simulink model "model_2D"  (R2021b)
settings: Solver=VariableStepAuto  StartTime=0.0  StopTime=discretization_time  RelTol=1e-3
values from neighbouring files (symbols this model uses):
  state = current_state+[0.5*time_step^2*input+current_state(2)*time_step,time_step*input]    [Model_1D.m]    (also in Model_der_1D.m = [1,time_step;0,1]; Model_der_2D.m = [1,0,-sin(current_state(3))*0.5*(current_state(5)+current_st; Model_obs_1D.m = [1,0;0,1]; Model_obs_2D.m = [1,0,0,0,0;0,1,0,0,0;0,0,1,0,0;0,0,0,1,0;0,0,0,0,1])
settings Model: Creator=filip  LastModifiedBy=filip

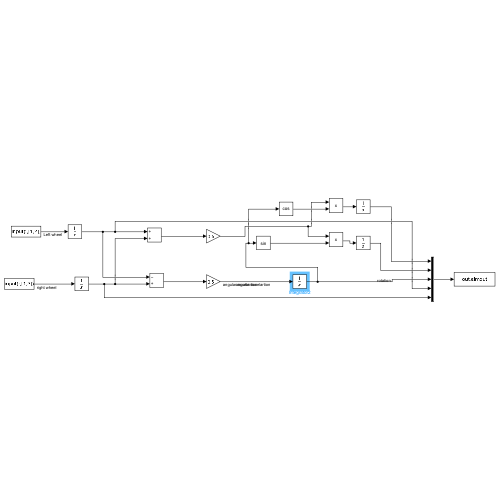
[thumbnail: Simulink's stored preview of the top-level diagram]
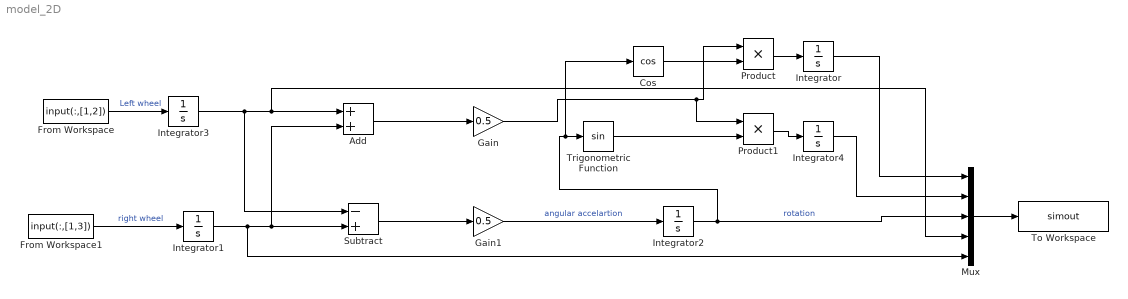
== system model_2D ==
  Add : Sum
  Cos : Trigonometry  Operator=cos
  From Workspace : FromWorkspace  VariableName=input(:,[1,2])
  From Workspace1 : FromWorkspace  VariableName=input(:,[1,3])
  Gain : Gain  Gain=0.5
  Gain1 : Gain  Gain=0.5
  Integrator : Integrator  InitialCondition=state(1)
  Integrator1 : Integrator  InitialCondition=state(5)
  Integrator2 : Integrator  InitialCondition=state(3)
  Integrator3 : Integrator  InitialCondition=state(4)
  Integrator4 : Integrator  InitialCondition=state(2)
  Mux : Mux  Inputs=5
  Product : Product
  Product1 : Product
  Subtract : Sum  Inputs=-+
  To Workspace : ToWorkspace  VariableName=simout  SaveFormat=Timeseries  SampleTime=-1
  Trigonometric Function : Trigonometry
  wires:
  From Workspace/1 -> Integrator3/1  "Left wheel"
  From Workspace1/1 -> Integrator1/1  "right wheel"
  Add/1 -> Gain/1
  Subtract/1 -> Gain1/1
  Gain1/1 -> Integrator2/1  "angular accelartion"
  Mux/1 -> To Workspace/1
  Integrator2/1 -> Mux/3, Cos/1, Trigonometric Function/1  "rotation"
  Integrator/1 -> Mux/1
  Integrator4/1 -> Mux/2
  Product/1 -> Integrator/1
  Product1/1 -> Integrator4/1
  Trigonometric Function/1 -> Product1/2
  Cos/1 -> Product/2
  Gain/1 -> Product1/1, Product/1
  Integrator3/1 -> Subtract/1, Mux/4, Add/1
  Integrator1/1 -> Mux/5, Subtract/2, Add/2
